simulink model "BloquesXY"  (R2016a)
settings: Solver=VariableStepAuto  StartTime=0.0  StopTime=10.0  RelTol=1e-3
libraries: simulink x1
settings Model: Creator=Marcelo  LastModifiedBy=Marcelo

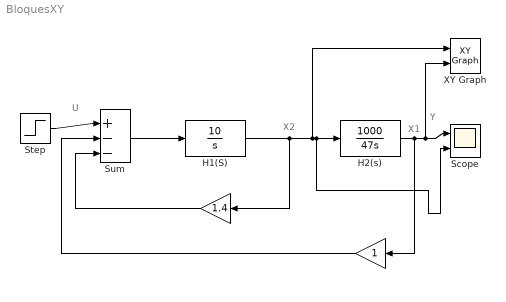
== system BloquesXY ==
  note: U
  note: Y
  note: X1
  note: X2
  " " : Gain
  " " : Gain  Gain=1.4
  H1(S) : TransferFcn  Numerator=[10]  Denominator=[1 0]
  H2(s) : TransferFcn  Numerator=[1000]  Denominator=[47 0]
  Scope : Scope  NumInputPorts=2
  Step : Step  After=4  SampleTime=0
  Sum : Sum  Inputs=|+--
  XY Graph : simulink/Sinks/XY Graph  xmin=-1  xmax=3  ymin=-1  ymax=5  st=0.01
  wires:
  Step/1 -> Sum/1
  Sum/1 -> H1(S)/1
  H2(s)/1 -> XY Graph/2, Scope/1, " "/1
  " "/1 -> Sum/3
  " "/1 -> Sum/2
  H1(S)/1 -> " "/1, XY Graph/1, Scope/2, H2(s)/1
